simulink model "Simulator_Case_3"  (R2024a)
settings: Solver=VariableStepAuto  StartTime=0.0  StopTime=100  RelTol=1e-3
values from neighbouring files (symbols this model uses):
  Time_Period_Sampling = 0.1    [Parametrization_Simulation_Case_3.m]
undefined symbols (not defined in the file or in its folder): Controller_PDF_Classical_Discrete, Damping_Factor_Waves, Pulsation_Wave, Rudder_To_Heading_Discretized, Static_Gain_Nomoto, Time_Constant_Total, Wave_Transfer_Function_Discrete
libraries: simulink_extras x2
settings Model: Creator=gerar  LastModifiedBy=gerar

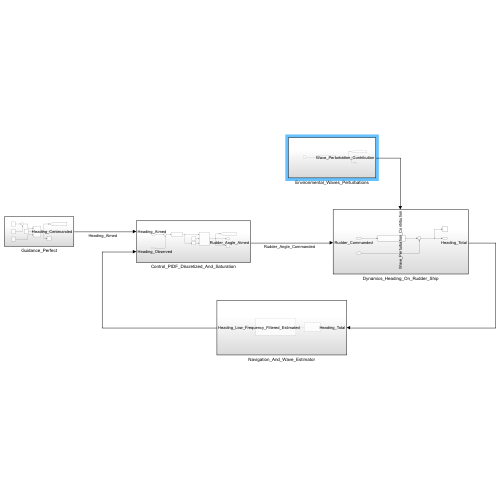
[thumbnail: Simulink's stored preview of the top-level diagram]
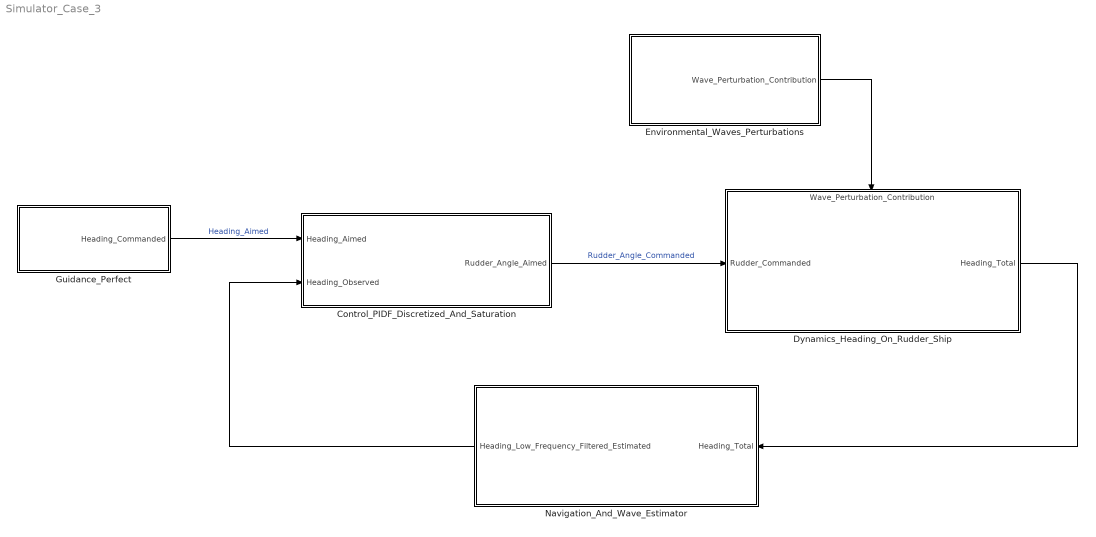
== system Simulator_Case_3 ==
  Control_PIDF_Discretized_And_Saturation : Subsystem
  Dynamics_Heading_On_Rudder_Ship : Subsystem
      settings: PortSchema="{\"entries\":[{\"content\":{\"sides\":[{\"content\":{\"connectorIds\":[\"In1\"]},\"type\":\"ConnectorPlacement.EquallySpacedRectSide\",\"uuid\":\"1262d93f-9737-49c5-b1c8-13d3f825160d\"},{\"content\":{\"connectorIds\":[\"Out1\"],\"side\":\"RIGHT\"},\"type\":\"ConnectorPlacement.EquallySpacedRectSide\",\"uuid\":\"2783823e-17f0-4da0-9b4a-e84aa912eb5f\"},{\"content\":{\"connectorIds\":[\"In2\"],\"side\":\"TOP\"},\"type\":\"ConnectorPlacement.EquallySpacedRectSide\",\"uuid\":\"9227960a-c500-4bd1-9392-f2e1de824969\"}]},\"type\":\"ConnectorPlacement.EquallySpacedConnector\",\"uuid\":\"fe1a7a14-057d-49da-982c-994c0d128614\"}],\"packageUris\":[\"http://schema.mathworks.com/mf0/Connector/R2020b\"],\"version\":\"1.0\"}"
  Environmental_Waves_Perturbations : Subsystem
  Guidance_Perfect : Subsystem
  Navigation_And_Wave_Estimator : Subsystem
  wires:
  Guidance_Perfect/1(Heading_Commanded) -> Control_PIDF_Discretized_And_Saturation/1(Heading_Aimed)  "Heading_Aimed"
  Navigation_And_Wave_Estimator/1(Heading_Low_Frequency_Filtered_Estimated) -> Control_PIDF_Discretized_And_Saturation/2(Heading_Observed)
  Control_PIDF_Discretized_And_Saturation/1(Rudder_Angle_Aimed) -> Dynamics_Heading_On_Rudder_Ship/1(Rudder_Commanded)  "Rudder_Angle_Commanded"
  Environmental_Waves_Perturbations/1(Wave_Perturbation_Contribution) -> Dynamics_Heading_On_Rudder_Ship/2(Wave_Perturbation_Contribution)
  Dynamics_Heading_On_Rudder_Ship/1(Heading_Total) -> Navigation_And_Wave_Estimator/1(Heading_Total)

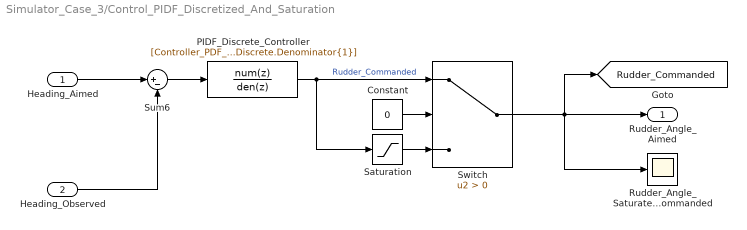
== system Simulator_Case_3/Control_PIDF_Discretized_And_Saturation ==
  Heading_Aimed : Inport
  Heading_Observed : Inport  Port=2
  Constant : Constant  Value=0
  PIDF_Discrete_Controller : DiscreteTransferFcn  Numerator=[Controller_PDF_Classical_Discrete.Numerator{1}]  Denominator=[Controller_PDF_Classical_Discrete.Denominator{1}]
  Rudder_Angle_Saturated_Commanded : Scope
  Saturation : Saturate  UpperLimit=35*(pi/180)  LowerLimit=-35*(pi/180)
  Sum6 : Sum  Inputs=|+-
  Switch : Switch  Criteria=u2 > Threshold  SaturateOnIntegerOverflow=off  InputSameDT=off
  Rudder_Angle_Aimed : Outport
  tag scope: Rudder_Commanded=global
  wires:
  Sum6/1 -> PIDF_Discrete_Controller/1
  Heading_Aimed/1 -> Sum6/1
  Heading_Observed/1 -> Sum6/2
  PIDF_Discrete_Controller/1 -> Saturation/1, Switch/1  "Rudder_Commanded"
  Constant/1 -> Switch/2
  Saturation/1 -> Switch/3
  Switch/1 -> Rudder_Angle_Saturated_Commanded/1, [Rudder_Commanded], Rudder_Angle_Aimed/1

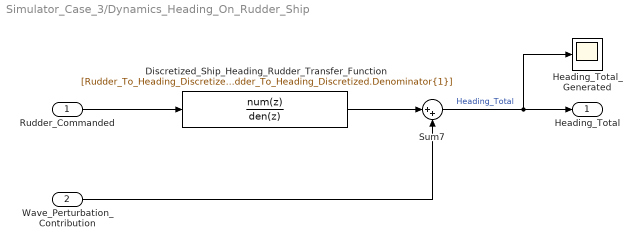
== system Simulator_Case_3/Dynamics_Heading_On_Rudder_Ship ==
  Rudder_Commanded : Inport
  Wave_Perturbation_Contribution : Inport  Port=2
  Discretized_Ship_Heading_Rudder_Transfer_Function : DiscreteTransferFcn  Numerator=[Rudder_To_Heading_Discretized.Numerator{1}]  Denominator=[Rudder_To_Heading_Discretized.Denominator{1}]
  Heading_Total_Generated : Scope
  Sum7 : Sum  Inputs=|++
  Heading_Total : Outport
  wires:
  Discretized_Ship_Heading_Rudder_Transfer_Function/1 -> Sum7/1
  Wave_Perturbation_Contribution/1 -> Sum7/2
  Rudder_Commanded/1 -> Discretized_Ship_Heading_Rudder_Transfer_Function/1
  Sum7/1 -> Heading_Total/1, Heading_Total_Generated/1  "Heading_Total"

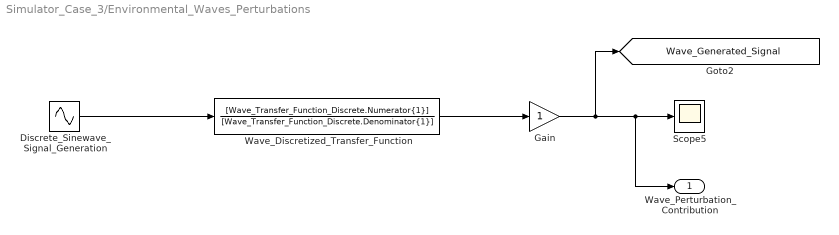
== system Simulator_Case_3/Environmental_Waves_Perturbations ==
  Discrete_Sinewave_Signal_Generation : Sin  Amplitude=1*(pi/180)  Frequency=Pulsation_Wave  SampleTime=Time_Period_Sampling
  Gain : Gain
  Scope5 : Scope
  Wave_Discretized_Transfer_Function : DiscreteTransferFcn  Numerator=[Wave_Transfer_Function_Discrete.Numerator{1}]  Denominator=[Wave_Transfer_Function_Discrete.Denominator{1}]
  Wave_Perturbation_Contribution : Outport
  tag scope: Wave_Generated_Signal=global
  wires:
  Gain/1 -> Wave_Perturbation_Contribution/1, Scope5/1, [Wave_Generated_Signal]
  Wave_Discretized_Transfer_Function/1 -> Gain/1
  Discrete_Sinewave_Signal_Generation/1 -> Wave_Discretized_Transfer_Function/1

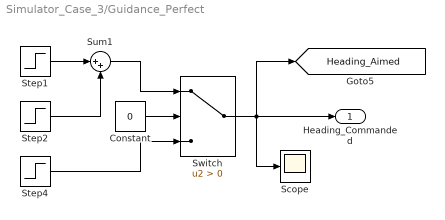
== system Simulator_Case_3/Guidance_Perfect ==
  Constant : Constant  Value=0
  Scope : Scope
  Step1 : Step  After=15*(pi/180)  SampleTime=0
  Step2 : Step  Time=5  After=22*(pi/180)  SampleTime=0
  Step4 : Step  After=30*(pi/180)  SampleTime=0
  Sum1 : Sum  Inputs=|++
  Switch : Switch  Criteria=u2 > Threshold  SaturateOnIntegerOverflow=off  InputSameDT=off
  Heading_Commanded : Outport
  tag scope: Heading_Aimed=global
  wires:
  Sum1/1 -> Switch/1
  Step2/1 -> Sum1/2
  Step1/1 -> Sum1/1
  Switch/1 -> Scope/1, [Heading_Aimed], Heading_Commanded/1
  Step4/1 -> Switch/3
  Constant/1 -> Switch/2

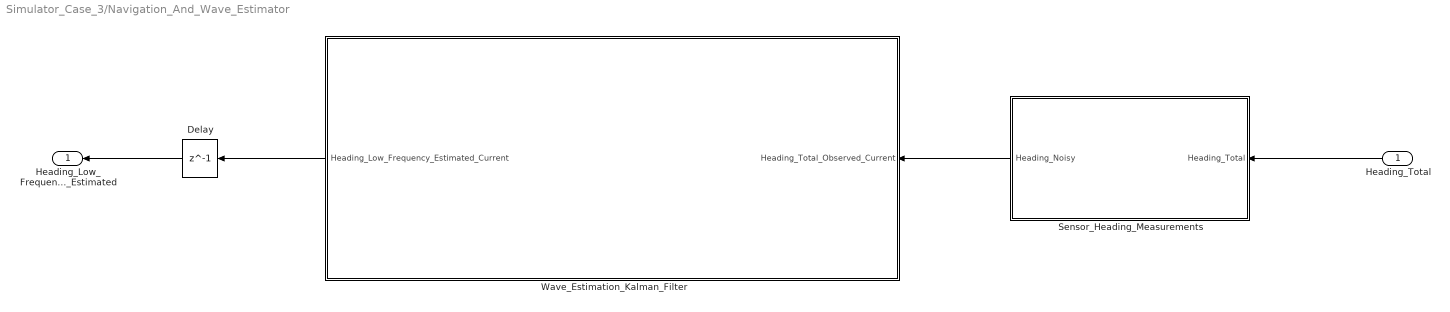
== system Simulator_Case_3/Navigation_And_Wave_Estimator ==
  Heading_Total : Inport
  Delay : Delay  DelayLength=1  InputProcessing=Columns as channels (frame based)
  Sensor_Heading_Measurements : Subsystem
  Wave_Estimation_Kalman_Filter : Subsystem
  Heading_Low_Frequency_Filtered_Estimated : Outport
  wires:
  Heading_Total/1 -> Sensor_Heading_Measurements/1(Heading_Total)
  Sensor_Heading_Measurements/1(Heading_Noisy) -> Wave_Estimation_Kalman_Filter/1(Heading_Total_Observed_Current)
  Wave_Estimation_Kalman_Filter/1(Heading_Low_Frequency_Estimated_Current) -> Delay/1
  Delay/1 -> Heading_Low_Frequency_Filtered_Estimated/1

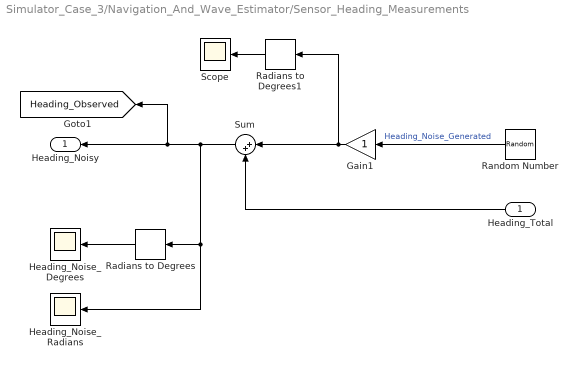
== system Simulator_Case_3/Navigation_And_Wave_Estimator/Sensor_Heading_Measurements ==
  Heading_Total : Inport
  Gain1 : Gain
  Heading_Noise_Degrees : Scope
  Heading_Noise_Radians : Scope
  Radians to Degrees : simulink_extras/Transformations/Radians to Degrees
  Radians to Degrees1 : simulink_extras/Transformations/Radians to Degrees
  Random Number : RandomNumber  Variance=((1*(pi/180))/3)^2  SampleTime=Time_Period_Sampling
  Scope : Scope
  Sum : Sum  Inputs=|++
  Heading_Noisy : Outport
  tag scope: Heading_Observed=global
  wires:
  Random Number/1 -> Gain1/1  "Heading_Noise_Generated"
  Radians to Degrees/1 -> Heading_Noise_Degrees/1
  Gain1/1 -> Radians to Degrees1/1, Sum/1
  Heading_Total/1 -> Sum/2
  Sum/1 -> Radians to Degrees/1, Heading_Noise_Radians/1, [Heading_Observed], Heading_Noisy/1
  Radians to Degrees1/1 -> Scope/1

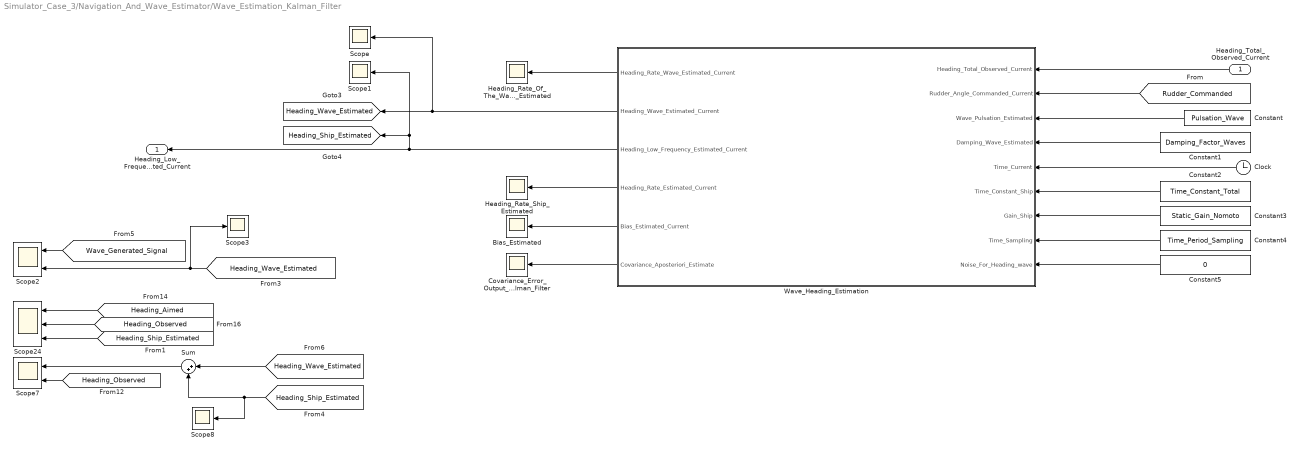
== system Simulator_Case_3/Navigation_And_Wave_Estimator/Wave_Estimation_Kalman_Filter ==
  Heading_Total_Observed_Current : Inport
  Bias_Estimated : Scope
  Clock : Clock
  Constant : Constant  Value=Pulsation_Wave  SampleTime=Time_Period_Sampling
  Constant1 : Constant  Value=Damping_Factor_Waves  SampleTime=Time_Period_Sampling
  Constant2 : Constant  Value=Time_Constant_Total  SampleTime=Time_Period_Sampling
  Constant3 : Constant  Value=Static_Gain_Nomoto  SampleTime=Time_Period_Sampling
  Constant4 : Constant  Value=Time_Period_Sampling  SampleTime=Time_Period_Sampling
  Constant5 : Constant  Value=0
  Covariance_Error_Output_Kalman_Filter : Scope
  Heading_Rate_Of_The_Waves_Estimated : Scope
  Heading_Rate_Ship_Estimated : Scope
  Scope{,1,3,8} (4 alike) : Scope
  Scope2 : Scope  NumInputPorts=2
  Scope24 : Scope  NumInputPorts=3
  Scope7 : Scope  NumInputPorts=2
  Sum : Sum  Inputs=|++
  Wave_Heading_Estimation : MATLAB Function  TreatAsAtomicUnit=on  SystemSampleTime=Time_Period_Sampling
  Heading_Low_Frequency_Estimated_Current : Outport
  tag scope: Heading_Ship_Estimated=global, Heading_Wave_Estimated=global
  wires:
  Wave_Heading_Estimation/3(Heading_Low_Frequency_Estimated_Current) -> Scope1/1, [Heading_Ship_Estimated], Heading_Low_Frequency_Estimated_Current/1
  Heading_Total_Observed_Current/1 -> Wave_Heading_Estimation/1(Heading_Total_Observed_Current)
  [Rudder_Commanded] -> Wave_Heading_Estimation/2(Rudder_Angle_Commanded_Current)
  Constant/1 -> Wave_Heading_Estimation/3(Wave_Pulsation_Estimated)
  Constant1/1 -> Wave_Heading_Estimation/4(Damping_Wave_Estimated)
  Clock/1 -> Wave_Heading_Estimation/5(Time_Current)
  Constant2/1 -> Wave_Heading_Estimation/6(Time_Constant_Ship)
  Constant3/1 -> Wave_Heading_Estimation/7(Gain_Ship)
  Constant4/1 -> Wave_Heading_Estimation/8(Time_Sampling)
  Constant5/1 -> Wave_Heading_Estimation/9(Noise_For_Heading_wave)
  Wave_Heading_Estimation/1(Heading_Rate_Wave_Estimated_Current) -> Heading_Rate_Of_The_Waves_Estimated/1
  Wave_Heading_Estimation/2(Heading_Wave_Estimated_Current) -> Scope/1, [Heading_Wave_Estimated]
  Wave_Heading_Estimation/5(Bias_Estimated_Current) -> Bias_Estimated/1
  Wave_Heading_Estimation/4(Heading_Rate_Estimated_Current) -> Heading_Rate_Ship_Estimated/1
  Wave_Heading_Estimation/6(Covariance_Aposteriori_Estimate) -> Covariance_Error_Output_Kalman_Filter/1
  [Heading_Wave_Estimated] -> Scope3/1, Scope2/2
  [Wave_Generated_Signal] -> Scope2/1
  [Heading_Observed] -> Scope24/2
  [Heading_Aimed] -> Scope24/1
  Sum/1 -> Scope7/1
  [Heading_Ship_Estimated] -> Scope8/1, Sum/2
  [Heading_Observed] -> Scope7/2
  [Heading_Wave_Estimated] -> Sum/1
  [Heading_Ship_Estimated] -> Scope24/3

== matlab function Simulator_Case_3/Navigation_And_Wave_Estimator/Wave_Estimation_Kalman_Filter/Wave_Heading_Estimation ==
  data: Heading_Total_Observed_Current input; Rudder_Angle_Commanded_Current input; Wave_Pulsation_Estimated input; Damping_Wave_Estimated input; Time_Current input; Time_Constant_Ship input; Gain_Ship input; Time_Sampling input; Noise_For_Heading_wave input; Heading_Rate_Wave_Estimated_Current output; Heading_Wave_Estimated_Current output; Heading_Low_Frequency_Estimated_Current output; Heading_Rate_Estimated_Current output; Bias_Estimated_Current output; Covariance_Aposteriori_Estimate output
function [Heading_Rate_Wave_Estimated_Current,...
          Heading_Wave_Estimated_Current,...
          Heading_Low_Frequency_Estimated_Current,...
          Heading_Rate_Estimated_Current,...
          Bias_Estimated_Current,...
          Covariance_Aposteriori_Estimate]= Kalman_Filter_Wave_Estimation(Heading_Total_Observed_Current,...
                                                                          Rudder_Angle_Commanded_Current,...
                                                                          Wave_Pulsation_Estimated,...
                                                                          Damping_Wave_Estimated,...
                                                                          Time_Current,...
                                                                          Time_Constant_Ship,...
                                                                          Gain_Ship,...
                                                                          Time_Sampling,...
                                                                          Noise_For_Heading_wave)

% Persistents definition:
persistent State_Model_Prediction;
persistent Covariance_Prediction;
persistent Rudder_Angle_Commanded_Prev;

% Integration step to be aligned with the sampling
% frequency:
Time_Integration = Time_Sampling;

% State model definition:
% -----------------------                          
% State matrix 'A':
State_Matrix = [1 Time_Integration 0 0 0;
                -Time_Integration*Wave_Pulsation_Estimated^2 1-2*Damping_Wave_Estimated*Wave_Pulsation_Estimated*Time_Integration 0 0 0;
                0 0 1 Time_Integration 0;
                0 0 0 1-(Time_Integration/Time_Constant_Ship) Time_Integration;
                0 0 0 0 1];
            
% Input matrix 'B':
Input_Matrix = [0;0;0;(Time_Integration*Gain_Ship)/Time_Constant_Ship;0];

% Noise state matrix 'G':
Noise_State_Matrix = [0 0 0;
                      Time_Integration*Wave_Pulsation_Estimated^2 0 0;
                      0 0 0;
                      0 Time_Integration 0;
                      0 0 Time_Integration];


% State model covariance matrix 'Q': must be better estimated.
Sigma_Heading_Wave = (270*(pi/180))/3;
%Sigma_Heading_Wave = sqrt(250);
Sigma_Rate_Heading = (5*(pi/180))/3;
Sigma_Bias = (15*(pi/180))/3;
State_Model_Covariance_Matrix = diag([Sigma_Heading_Wave^2,Sigma_Rate_Heading^2,Sigma_Bias^2]);


% Measurement model definition:
% -----------------------------
Measurement_Matrix = [0 1 1 0 0];
% Measurement model covariance matrix 'R':
Sigma_Heading_Estimated = ((25*pi/180)/3); % Must be the same amount of noise applied in the heading in input of the filter (ie: sensor noise).
Measurement_Model_Covariance_Matrix = Sigma_Heading_Estimated^2;
Measurement_Vector_Current = Heading_Total_Observed_Current;

% Kalman filter equations:
% ------------------------
% Prediction:
% -----------
% State parameters propagation through the model for estimation:
if isempty(State_Model_Prediction)
    Heading_Rate_Wave_Model_Previous = 0;
    Heading_Wave_Model_Previous = 0;
    Heading_Low_Frequency_Model_Previous = 0;
    Heading_Rate_Model_Previous = 0;
    Bias_Model_Previous = 0;
    State_Model_Prediction = [Heading_Rate_Wave_Model_Previous;
                              Heading_Wave_Model_Previous;...
                              Heading_Low_Frequency_Model_Previous;...
                              Heading_Rate_Model_Previous;
                              Bias_Model_Previous];
end
if isempty(Rudder_Angle_Commanded_Prev)
    Rudder_Angle_Commanded_Prev = 0;
end
State_Vector_Model_Apriori_Estimated_Current = State_Matrix*State_Model_Prediction + Input_Matrix*Rudder_Angle_Commanded_Current;
% Predicted apriori estimated covariance:
if isempty(Covariance_Prediction)
    Covariance_Prediction = Noise_State_Matrix*State_Model_Covariance_Matrix*Noise_State_Matrix';
end
Predicted_Apriori_Estimated_Covariance_Previous = Covariance_Prediction;
Predicted_Apriori_Estimated_Covariance_Current = State_Matrix*Predicted_Apriori_Estimated_Covariance_Previous*State_Matrix' + ...
                                                 Noise_State_Matrix*State_Model_Covariance_Matrix*Noise_State_Matrix';

% Innovation:
Measurement_Innovation = Measurement_Vector_Current - Measurement_Matrix*State_Vector_Model_Apriori_Estimated_Current;
% Covariance:
Covariance_Innovation = Measurement_Matrix*Predicted_Apriori_Estimated_Covariance_Current*Measurement_Matrix' + Measurement_Model_Covariance_Matrix;
% Optimal Kalman gain:
Kalman_Gain = Predicted_Apriori_Estimated_Covariance_Current*Measurement_Matrix'*inv(Covariance_Innovation);
% A posteriori state estimate:
State_Vector_Aposteriori_Estimate = State_Vector_Model_Apriori_Estimated_Current + Kalman_Gain*Measurement_Innovation;
% A posteriori estimate covariance:
Covariance_Aposteriori_Estimate = (eye(size(Kalman_Gain*Measurement_Matrix,1)) - Kalman_Gain*Measurement_Matrix)*Predicted_Apriori_Estimated_Covariance_Current;

% Update the outputs:
Heading_Rate_Wave_Estimated_Current = State_Vector_Aposteriori_Estimate(1);
Heading_Wave_Estimated_Current = State_Vector_Aposteriori_Estimate(2);
Heading_Low_Frequency_Estimated_Current = State_Vector_Aposteriori_Estimate(3);
Heading_Rate_Estimated_Current = State_Vector_Aposteriori_Estimate(4);
Bias_Estimated_Current = State_Vector_Aposteriori_Estimate(5);

% Update the Kalman Filter states and covariance for the next prediction:
State_Model_Prediction = State_Vector_Aposteriori_Estimate;
Covariance_Prediction = Covariance_Aposteriori_Estimate;
Rudder_Angle_Commanded_Prev = Rudder_Angle_Commanded_Current;

end
